simulink model "FactorialStateFlow"  (R2020a)
settings: Solver=FixedStepDiscrete  StartTime=0.0  StopTime=10.0  RelTol=1e-3
settings Model: Creator=yomna  LastModifiedBy=yomna
settings OptimizationCC: DefaultParameterBehavior=Inlined  EnhancedBackFolding=on  PassReuseOutputArgsAs=Individual arguments  ZeroExternalMemoryAtStartup=off  ZeroInternalMemoryAtStartup=off  OptimizeBlockOrder=speed  DifferentSizesBufferReuse=on  OptimizationCustomize=off  EfficientTunableParamExpr=on
settings DebuggingCC: UnderspecifiedInitializationDetection=Classic  MergeDetectMultiDrivingBlocksExec=none  ParameterTunabilityLossMsg=error
settings ModelReferenceCC: PropagateSignalLabelsOutOfModel=off
settings SFSimCC: MATLABDynamicMemAlloc=off
settings RTWCC: SystemTargetFile=ert.tlc  GenCodeOnly=on  TemplateMakefile=ert_default_tmf  GenerateReport=on  IncludeHyperlinkInReport=on  LaunchReport=on  GenerateTraceInfo=on  GenerateTraceReport=on  GenerateTraceReportSl=on  GenerateTraceReportSf=on  GenerateTraceReportEml=on
settings CodeAppCC: ForceParamTrailComments=on  IgnoreCustomStorageClasses=off  OperatorAnnotations=on  SimulinkDataObjDesc=on  SFDataObjDesc=on  InsertBlockDesc=on
settings ERTTargetCC: TargetLangStandard=C99 (ISO)  GenerateSampleERTMain=on  InlinedParameterPlacement=NonHierarchical  ERTCustomFileTemplate=example_file_process.tlc

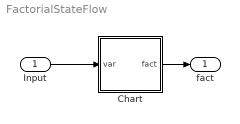
== system FactorialStateFlow ==
  Input : Inport
  Chart : Stateflow chart  TreatAsAtomicUnit=on
  fact : Outport
  wires:
  Chart/1(fact) -> fact/1
  Input/1 -> Chart/1(var)

== stateflow chart FactorialStateFlow/Chart ==
  (default) -> (junction 8)
  (junction 8) -> (junction 10) : {fact=1; counter=var;}
  (junction 10) -> (junction 9) [order 1] : [counter>1]
  (junction 12) -> (junction 10)
  (junction 9) -> (junction 11) : {fact=fact*counter}
  (junction 10) -> (junction 13) [order 2]
  (junction 11) -> (junction 12) : {counter = counter - 1;}
  data: var input uint8; fact output uint32; counter local uint8
